simulink model "dspilbclib"  (R2020a)
settings: Solver=FixedStepDiscrete  StartTime=0.0  StopTime=inf  RelTol=1e-3  EnableMultiTasking=on
InitFcn:
  | ilbcDatatype = get_param([bdroot '/Configuration'],'ilbcDialogDatatype');
  | if strcmp(get_param([bdroot '/Configuration'],'ilbcDialogMode'), '13.33 kbit/sec mode')
  |   ilbcMode = 1;
  | else
  |   ilbcMode = 2;
  | end
model workspace: external: MAT-File dspilbcdata.mat (data not in the file)
undefined symbols (not defined in the file or in its folder): ilbc, Newton, Raphson
libraries: simulink x33, dspmtrx3 x28, dspquant2 x9, dspilbclib x8, dspstat3 x8, dspsigops x7, simulink_need_slupdate x3, dspsrcs4 x2, dspsnks4 x1, dspvision x1, dspmisc x1, dsplp x1
(part 1 of 3)
CloseFcn:
  | clear ilbcMode;
  | clear ilbcDatatype
settings Model: ExtModeAutoUpdateStatusClock=off  Creator=The MathWorks, Inc.  LastModifiedBy=Bs Computer
settings DataIOCC: LimitDataPoints=on  SaveFormat=Array  SaveOutput=off  SignalLogging=off  SaveTime=off  ReturnWorkspaceOutputs=off
settings OptimizationCC: DefaultParameterBehavior=Inlined  ExpressionDepthLimit=2147483647  InitFltsAndDblsToZero=on  EfficientFloat2IntCast=on  EfficientMapNaN2IntZero=off  LifeSpan=inf  SimCompilerOptimization=on
settings DebuggingCC: UnderspecifiedInitializationDetection=Classic  MergeDetectMultiDrivingBlocksExec=none  SolverPrmCheckMsg=warning  InheritedTsInSrcMsg=none  SigSpecEnsureSampleTimeMsg=none  Int32ToFloatConvMsg=none  ParameterPrecisionLossMsg=none  FcnCallInpInsideContextMsg=warning  AllowSymbolicDim=off  StateNameClashWarn=warning  StrictBusMsg=ErrorOnBusTreatedAsVector  SFUnexpectedBacktrackingDiag=warning  SFNoUnconditionalDefaultTransitionDiag=warning  SFExecutionAtInitializationDiag=none  ArithmeticOperatorsInVariantConditions=warning
settings HardwareCC: ProdBitPerPointer=32  ProdBitPerSizeT=32  ProdBitPerPtrDiffT=32  ProdLargestAtomicFloat=None  ProdIntDivRoundTo=Floor  ProdEndianess=Unspecified  ProdWordSize=32  ProdHWDeviceType=32-bit Generic
settings ModelReferenceCC: UpdateModelReferenceTargets=IfOutOfDate  PropagateSignalLabelsOutOfModel=off
settings SFSimCC: SimUseLocalCustomCode=off  SimParseCustomCode=off  CustomCodeUndefinedFunction=UseInterfaceOnly
settings RTWCC: RTWUseLocalCustomCode=off
settings CodeAppCC: StateflowObjectComments=on
settings GRTTargetCC: TargetFcnLib=ansi_tfl_tmw_new.mat  TargetLangStandard=C89/C90 (ANSI)  CombineOutputUpdateFcns=off  GRTInterface=on
settings ConfigComp: CovMetricSettings=dw  CovHtmlReporting=on  CovSaveCumulativeToWorkspaceVar=on  CovSaveSingleToWorkspaceVar=on  CovExternalEMLEnable=off  CovSFcnEnable=off

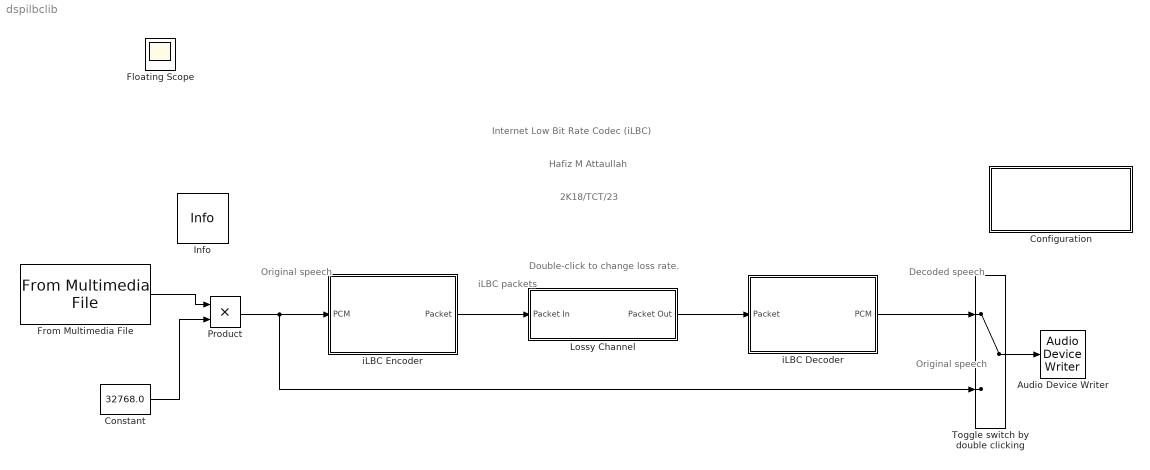
== system dspilbclib ==
  note: Internet Low Bit Rate Codec (iLBC)
  note: Original
      | speech
  note: iLBC
      | packets
  note: Double-click to change loss rate.
  note: Decoded
      | speech
  note: Original
      | speech
  note: 2K18/TCT/23
  note: Hafiz M Attaullah
  Audio Device Writer : dspsnks4/Audio Device Writer  Driver=DirectSound  Device=Default  InheritSampleRate=on  SampleRate=44100  BitDepth=16-bit integer  BufferSize=4096  NumBuffers=10  DefaultOutputChannelMapping=on  OutputChannelMapping=1:2  OutputNumUnderrunSamples=off  DriverIdx=1  DeviceWarnFlag=''
  Configuration : Subsystem  mask(iLBC Configuration){ilbcDialogMode=13.33 kbit/sec mode, ilbcDialogDatatype=double}
      mask prompts: ilbcDialogMode "iLBC mode:"; ilbcDialogDatatype "Internal data type:"
      mask help:
      | The iLBC standard is defined for two data rates: 13.33 kbit/sec and 15.20 kbit/sec.  Running under 13.33 kbit/sec, the encoder creates and outputs a compressed speech packet every 30ms.  With the 15.20 kbit/sec data rate, the encoder will output a packet every 20ms.  For the 13.33 kbit/sec mode, the packet size is a uint8 column vector of length 50, where each element represents one byte.  For the 15.20 kbit/sec mode, the packet is of length 38 bytes.
      |
      | The "Internal Data Type" option controls the precision for all internal floating point calculations in the iLBC Encoder and Decoder. The possible options are double and single precision.
      mask init:
      | if ilbcDialogMode == 1
      |     ilbcModeStr = '13.33';
      | elseif ilbcDialogMode == 2
      |     ilbcModeStr = '15.20';
      | end
      | 
      | if ilbcDialogDatatype == 1
      |     ilbcDatatype = 'double';
      | elseif ilbcDialogDatatype == 2
      |     ilbcDatatype = 'single';
      | end
      mask TypeOptions ilbcDialogMode: 13.33 kbit/sec mode | 15.20 kbit/sec mode
      mask TypeOptions ilbcDialogDatatype: double | single
      mask Display:
      | disp([ilbcModeStr ' kb/sec mode\n' ...
      |     'Internal data type: ' ilbcDatatype '\n' ...
      |     '[Double-click to change]']);
  Constant : Constant  Value=32768.0
  From Multimedia File : dspvision/From Multimedia File  inputFilename=speech_dft_8kHz.wav  readRange=[1 Inf]  loop=on  numPlays=inf  outputStreams=Audio only  videoDataType=single  audioDataType=double  inheritSampleTime=on  userDefinedSampleTime=1/30  noAudioOutput=off  isIntensityVideo=off  fourcc=RGB  colorVideoFormat=Separate color signals  outputEOF=off  dataOrg=Column-major  audioFrameSize=ilbc.BLOCKL{ilbcMode}  computeAudioFrameSize=off  outSamplingMode=Sample based
  Info : dspmisc/Info  SystemSampleTime=-1  Latency=0  AutoFrameSizeCalculation=off
      settings: SourceProductBaseCode=DS
  Lossy Channel : Subsystem  TreatAsAtomicUnit=on  mask(Lossy Channel){PercentLoss=3}
      mask prompts: PercentLoss "Percent of Packets Lost (0-100)"
      mask help:
      | This subsystem simulates a lossy channel by setting a specified percentage of packets to all zeros.  Enter the percentage of packets to be lost as a number in the range 0-100.
      |
      | Note that the packet loss concealment algorithm in the iLBC Decoder is tuned for packet loss rates between 0-10%.  Loss rates above 10% will result in decoded speech with clearly audible errors.
      mask Display: disp([num2str(PercentLoss) '% Random Packet Loss']);
  Product : Product  OutDataTypeStr=int16
  Toggle switch by double clicking : ManualSwitch
  iLBC Decoder : Subsystem  TreatAsAtomicUnit=on
  iLBC Encoder : Subsystem  TreatAsAtomicUnit=on
  Floating Scope : Scope
  wires:
  iLBC Encoder/1(Packet) -> Lossy Channel/1(Packet In)
  Toggle switch by double clicking/1 -> Audio Device Writer/1
  Lossy Channel/1(Packet Out) -> iLBC Decoder/1(Packet)
  iLBC Decoder/1(PCM) -> Toggle switch by double clicking/1
  Constant/1 -> Product/2
  From Multimedia File/1 -> Product/1
  Product/1 -> Toggle switch by double clicking/2, iLBC Encoder/1(PCM)

== system dspilbclib/Configuration ==

== system dspilbclib/Lossy Channel ==
  Packet In : Inport
  Compare To Constant : simulink/Logic and Bit Operations/Compare To Constant  relop=>  const=PercentLoss  OutDataTypeStr=uint8  ZeroCross=off
  Gain : Gain  Gain=0  OutDataTypeStr=Inherit: Same as input
  Multiport Switch : MultiPortSwitch  DataPortOrder=Zero-based contiguous  Inputs=2  zeroidx=on
  Random Source : dspsrcs4/Random Source  SrcType=Uniform  NormMethod=Ziggurat  CltLength=12  MinVal=0  MaxVal=100  MeanVal=0  VarVal=1  RepMode=Not repeatable  rawSeed=1  IsInherit=off  SampMode=Discrete  SampTime=-1  SampFrame=1  DataType=Single  OutComplex=Real  OutputFrames=on
  Packet Out : Outport
  wires:
  Multiport Switch/1 -> Packet Out/1
  Random Source/1 -> Compare To Constant/1
  Compare To Constant/1 -> Multiport Switch/1
  Packet In/1 -> Multiport Switch/3, Gain/1
  Gain/1 -> Multiport Switch/2

== system dspilbclib/iLBC Decoder ==
  note: Section 4 of the iLBC standard
  Packet : Inport
  Data Type Duplicate : DataTypeDuplicate
  Data Type Duplicate1 : DataTypeDuplicate
  Data Type Conversion : DataTypeConversion  OutDataTypeStr=int16  SaturateOnIntegerOverflow=on
  Decode Sub-Blocks (4.1 - 4.4) : Subsystem
  Delay1 : Delay  DelayLength=1  InitialCondition=0
  Delay2 : Delay  DelayLength=1  InitialCondition=0
  Enable PLC : Constant  OutDataTypeStr=boolean
  High Pass Filter (4.8) : DiscreteFilter  Numerator=ilbc.hpo_zero_coefsTbl  Denominator=ilbc.hpo_pole_coefsTbl  InputProcessing=Columns as channels (frame based)  FilterStructure=Direct form II transposed  a0EqualsOne=on  NumAccumDataTypeStr=Inherit: Same as product output  DenAccumDataTypeStr=Inherit: Same as product output
  Logical Operator : Logic  AllPortsSameDT=off  OutDataTypeStr=boolean
  Logical Operator1 : Logic  Operator=NOT  AllPortsSameDT=off  OutDataTypeStr=boolean
  Multiport Switch : MultiPortSwitch  DataPortOrder=Zero-based contiguous  Inputs=2  zeroidx=on
  Multiport Switch1 : MultiPortSwitch  DataPortOrder=Zero-based contiguous  Inputs=2  zeroidx=on
  Packet Loss Concealment (4.5) : Subsystem
  Saturation : Saturate  UpperLimit=32767  LowerLimit=-32768
  Set data type to back-propagate : Constant  OutDataTypeStr=ilbcDatatype
  Split Packet (3.8) : Subsystem  TreatAsAtomicUnit=on
  Synthesis Filtering (4.7) : Subsystem  TreatAsAtomicUnit=on
  PCM : Outport
  wires:
  Enable PLC/1 -> Logical Operator/2
  Set data type to back-propagate/1 -> Data Type Duplicate/1
  Logical Operator1/1 -> Logical Operator/1
  Logical Operator/1 -> Packet Loss Concealment (4.5)/Enable
  Packet Loss Concealment (4.5)/2(Synthesis) -> Multiport Switch1/2
  Packet Loss Concealment (4.5)/1(Residual) -> Multiport Switch/2
  Decode Sub-Blocks (4.1 - 4.4)/2(Synthesis) -> Data Type Duplicate1/2, Multiport Switch1/3
  Decode Sub-Blocks (4.1 - 4.4)/1(Residual) -> Multiport Switch/3
  Split Packet (3.8)/8(Good Frame) -> Decode Sub-Blocks (4.1 - 4.4)/Enable, Multiport Switch1/1, Multiport Switch/1, Logical Operator1/1
  Split Packet (3.8)/1(Lsf Indices) -> Decode Sub-Blocks (4.1 - 4.4)/1(Lsf Indices)
  Split Packet (3.8)/7(Gain Indices) -> Decode Sub-Blocks (4.1 - 4.4)/7(Gain Indices)
  Split Packet (3.8)/6(Code Indices) -> Decode Sub-Blocks (4.1 - 4.4)/6(Code Indices)
  Split Packet (3.8)/5(Start State Indices) -> Decode Sub-Blocks (4.1 - 4.4)/5(Start State Indices)
  Split Packet (3.8)/4(Start State Gain Index) -> Decode Sub-Blocks (4.1 - 4.4)/4(Start State Gain Index)
  Split Packet (3.8)/3(State First) -> Decode Sub-Blocks (4.1 - 4.4)/3(State First)
  Split Packet (3.8)/2(Start State Number) -> Decode Sub-Blocks (4.1 - 4.4)/2(Start State Number)
  Synthesis Filtering (4.7)/1(Decoded Block) -> High Pass Filter (4.8)/1
  Saturation/1 -> Data Type Duplicate/2, Data Type Conversion/1
  Data Type Conversion/1 -> PCM/1
  Packet/1 -> Split Packet (3.8)/1(Packet)
  High Pass Filter (4.8)/1 -> Saturation/1
  Multiport Switch/1 -> Delay1/1, Synthesis Filtering (4.7)/1(Residual)
  Delay1/1 -> Packet Loss Concealment (4.5)/1(Last Residual)
  Multiport Switch1/1 -> Delay2/1, Data Type Duplicate1/1, Synthesis Filtering (4.7)/2(Synthesis Filters)
  Delay2/1 -> Packet Loss Concealment (4.5)/2(Last Synthesis)

== system dspilbclib/iLBC Encoder ==
  note: Section 3 of the iLBC standard
  PCM : Inport
  Calculate Residual (3.3) : Subsystem  TreatAsAtomicUnit=on
  Create Packet (3.8) : Subsystem  TreatAsAtomicUnit=on
  Data Type Conversion : DataTypeConversion  OutDataTypeStr=ilbcDatatype
  Encode Data (3.5 - 3.7) : Subsystem  TreatAsAtomicUnit=on
  Encoder LPC Analysis (3.2) : Subsystem  TreatAsAtomicUnit=on
  High Pass (3.1) : DiscreteFilter  Numerator=ilbc.hpi_zero_coefsTbl  Denominator=ilbc.hpi_pole_coefsTbl  InputProcessing=Columns as channels (frame based)  FilterStructure=Direct form II transposed  a0EqualsOne=on  NumAccumDataTypeStr=Inherit: Same as product output  DenAccumDataTypeStr=Inherit: Same as product output
  Perceptual Weighting (3.4) : dspmtrx3/Array-Vector Multiply  mode=Mute  saveAsFlag=0  Dimension=1  V_Source=Dialog parameter  V_VectFromMask=ilbc.LPC_CHIRP_WEIGHTDENUM.^(0:10)'  roundingMode=Floor  overflowMode=off  firstCoeffSignedness=Auto  firstCoeffDataTypeStr=Inherit: Same word length as input  firstCoeffMin=[]  firstCoeffMax=[]  firstCoeffLastDataTypeStr=Inherit: Same word length as input  prodOutputSignedness=Auto  accumSignedness=Auto  outputSignedness=Auto  outputDataTypeStr=Inherit: Same as product output  outputMin=[]  outputMax=[]  outputLastDataTypeStr=Inherit: Same as product output
      settings: SourceProductBaseCode=DS
  Packet : Outport
  wires:
  Data Type Conversion/1 -> High Pass (3.1)/1
  Encoder LPC Analysis (3.2)/1(LSF Indices) -> Create Packet (3.8)/1(LSF Indices)
  High Pass (3.1)/1 -> Calculate Residual (3.3)/2(Data), Encoder LPC Analysis (3.2)/1(Data)
  Encode Data (3.5 - 3.7)/6(Gain Indices) -> Create Packet (3.8)/7(Gain Indices)
  Encode Data (3.5 - 3.7)/5(Code Indices) -> Create Packet (3.8)/6(Code Indices)
  Encode Data (3.5 - 3.7)/4(Start State Indices) -> Create Packet (3.8)/5(Start State Indices)
  Encode Data (3.5 - 3.7)/3(Start State Gain Index) -> Create Packet (3.8)/4(Start State Gain Index)
  Encode Data (3.5 - 3.7)/2(State First) -> Create Packet (3.8)/3(State First)
  Encode Data (3.5 - 3.7)/1(Start State Number) -> Create Packet (3.8)/2(Start State Number)
  Encoder LPC Analysis (3.2)/3(Weight Filters) -> Perceptual Weighting (3.4)/1
  Calculate Residual (3.3)/1(Residual) -> Encode Data (3.5 - 3.7)/3(Residual)
  Create Packet (3.8)/1(Packet) -> Packet/1
  PCM/1 -> Data Type Conversion/1
  Perceptual Weighting (3.4)/1 -> Encode Data (3.5 - 3.7)/2(Weights)
  Encoder LPC Analysis (3.2)/2(Synthesis Filters) -> Calculate Residual (3.3)/1(Synthesis Filters), Encode Data (3.5 - 3.7)/1(Synthesis)

== system dspilbclib/iLBC Decoder/Decode Sub-Blocks (4.1 - 4.4) ==
  Lsf Indices : Inport
  Start State Number : Inport  Port=2
  State First : Inport  Port=3
  Start State Gain Index : Inport  Port=4
  Start State Indices : Inport  Port=5
  Code Indices : Inport  Port=6
  Gain Indices : Inport  Port=7
  Enable : EnablePort
  Decode Remaining Sub-Blocks (4.3 - 4.4) : Subsystem  TreatAsAtomicUnit=on
  Decode Start State : dspilbclib/Decode Start State  SystemSampleTime=-1  Latency=0  AutoFrameSizeCalculation=off
      settings: SourceProductBaseCode=DS
  Decoder LPC Analysis (4.1) : Subsystem  TreatAsAtomicUnit=on
  Selector1 : Selector  NumberOfDimensions=2  InputPortWidth=3  IndexOptions=Select all,Index vector (port)  Indices=-1,-1  OutputSizes=1
  Residual : Outport
  Synthesis : Outport  Port=2
  wires:
  Decode Start State/1 -> Decode Remaining Sub-Blocks (4.3 - 4.4)/1(Initial Codebook)
  Start State Number/1 -> Selector1/2, Decode Remaining Sub-Blocks (4.3 - 4.4)/4(Start State Number)
  Selector1/1 -> Decode Start State/3
  State First/1 -> Decode Start State/4, Decode Remaining Sub-Blocks (4.3 - 4.4)/5(State First)
  Lsf Indices/1 -> Decoder LPC Analysis (4.1)/1(LSF Indices)
  Decoder LPC Analysis (4.1)/1(Synthesis) -> Synthesis/1, Selector1/1
  Start State Indices/1 -> Decode Start State/1
  Start State Gain Index/1 -> Decode Start State/2
  Code Indices/1 -> Decode Remaining Sub-Blocks (4.3 - 4.4)/2(Code Indices)
  Gain Indices/1 -> Decode Remaining Sub-Blocks (4.3 - 4.4)/3(Gain Indices)
  Decode Remaining Sub-Blocks (4.3 - 4.4)/1(Residual) -> Residual/1

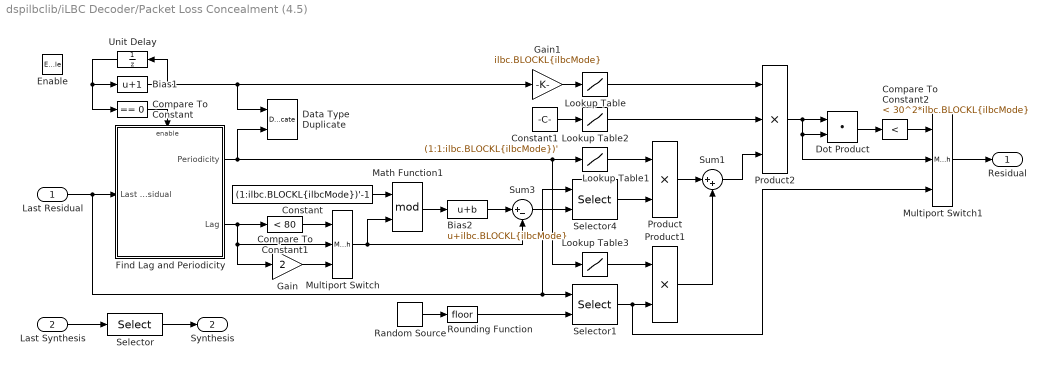
== system dspilbclib/iLBC Decoder/Packet Loss Concealment (4.5) ==
  Last Residual : Inport
  Last Synthesis : Inport  Port=2
  Enable : EnablePort  StatesWhenEnabling=reset
  Bias1 : Bias  Bias=1
  Bias2 : Bias  Bias=ilbc.BLOCKL{ilbcMode}
  Compare To Constant : simulink/Logic and Bit Operations/Compare To Constant  relop===  const=0  OutDataTypeStr=boolean  ZeroCross=off
  Compare To Constant1 : simulink/Logic and Bit Operations/Compare To Constant  relop=<  const=80  OutDataTypeStr=uint8  ZeroCross=off
  Compare To Constant2 : simulink/Logic and Bit Operations/Compare To Constant  relop=<  const=30^2*ilbc.BLOCKL{ilbcMode}  OutDataTypeStr=boolean  ZeroCross=off
  Constant : Constant  Value=(1:ilbc.BLOCKL{ilbcMode})'-1  VectorParams1D=off  OutDataTypeStr=Inherit: Inherit via back propagation
  Constant1 : Constant  Value=(1:1:ilbc.BLOCKL{ilbcMode})'  VectorParams1D=off  OutDataTypeStr=Inherit: Inherit via back propagation
  Data Type Duplicate : DataTypeDuplicate
  Dot Product : DotProduct  InputSameDT=on  OutDataTypeStr=Inherit: Inherit via internal rule
  Find Lag and Periodicity : Subsystem  TreatAsAtomicUnit=on
  Gain : Gain  Gain=2  OutDataTypeStr=Inherit: Same as input
  Gain1 : Gain  Gain=ilbc.BLOCKL{ilbcMode}  OutDataTypeStr=Inherit: Inherit via back propagation  ParamDataTypeStr=Inherit: Same as input
  Lookup Table : Lookup_n-D  NumberOfTableDimensions=1  BreakpointsForDimension1=[0 320 640 960 1280]  Table=[1.0 0.9 0.7 0.5 0.0]  InterpMethod=Flat  InputSameDT=on
  Lookup Table1 : Lookup_n-D  NumberOfTableDimensions=1  BreakpointsForDimension1=[0.3 0.6]  Table=[0 1]  ExtrapMethod=Clip  InputSameDT=on
  Lookup Table2 : Lookup_n-D  NumberOfTableDimensions=1  BreakpointsForDimension1=[80 160 240]  Table=[1.00 0.95 0.90]  ExtrapMethod=Clip  InputSameDT=on
  Lookup Table3 : Lookup_n-D  NumberOfTableDimensions=1  BreakpointsForDimension1=[0.3 0.6]  Table=[1 0]  ExtrapMethod=Clip  InputSameDT=on
  Math Function1 : Math  Operator=mod  SignedPower=on  SaturateOnIntegerOverflow=on
  Multiport Switch : MultiPortSwitch  DataPortOrder=Zero-based contiguous  Inputs=2  zeroidx=on
  Multiport Switch1 : MultiPortSwitch  DataPortOrder=Zero-based contiguous  Inputs=2  zeroidx=on
  Product : Product  RndMeth=Zero
  Product1 : Product  RndMeth=Zero
  Product2 : Product  Inputs=3  RndMeth=Zero  OutDataTypeStr=Inherit: Same as first input
  Random Source : dspsrcs4/Random Source  SrcType=Uniform  NormMethod=Ziggurat  CltLength=12  MinVal=ilbc.BLOCKL{ilbcMode}-70  MaxVal=ilbc.BLOCKL{ilbcMode}-0.001  MeanVal=0  VarVal=1  RepMode=Not repeatable  rawSeed=1  IsInherit=off  SampMode=Discrete  SampTime=-1  SampFrame=ilbc.BLOCKL{ilbcMode}  DataType=Single  OutComplex=Real  OutputFrames=off
  Rounding Function : Rounding
  Selector : Selector  NumberOfDimensions=2  InputPortWidth=3  IndexOptions=Select all,Index vector (dialog)  Indices=[1 3],repmat(ilbc.NSUB{ilbcMode},1,ilbc.NSUB{ilbcMode})  OutputSizes=1,1
  Selector1 : Selector  NumberOfDimensions=2  IndexMode=Zero-based  InputPortWidth=3  IndexOptions=Index vector (port),Select all  Indices=[1 3],1  OutputSizes=1,1
  Selector4 : Selector  NumberOfDimensions=2  IndexMode=Zero-based  InputPortWidth=3  IndexOptions=Index vector (port),Select all  Indices=[1 3],1  OutputSizes=1,1
  Sum1 : Sum  Inputs=|++
  Sum3 : Sum  Inputs=|+-
  Unit Delay : UnitDelay  SampleTime=-1  HasFrameUpgradeWarning=on
  Residual : Outport
  Synthesis : Outport  Port=2
  wires:
  Bias1/1 -> Data Type Duplicate/1, Gain1/1, Unit Delay/1
  Rounding Function/1 -> Selector1/2
  Unit Delay/1 -> Compare To Constant/1, Bias1/1
  Compare To Constant/1 -> Find Lag and Periodicity/Enable
  Random Source/1 -> Rounding Function/1
  Gain/1 -> Multiport Switch/3
  Product1/1 -> Sum1/2
  Product/1 -> Sum1/1
  Selector1/1 -> Multiport Switch1/3, Product1/2
  Lookup Table3/1 -> Product1/1
  Selector4/1 -> Product/2
  Lookup Table1/1 -> Product/1
  Multiport Switch/1 -> Sum3/2, Math Function1/2
  Sum3/1 -> Selector4/2
  Bias2/1 -> Sum3/1
  Math Function1/1 -> Bias2/1
  Constant/1 -> Math Function1/1
  Product2/1 -> Multiport Switch1/2, Dot Product/2, Dot Product/1
  Last Residual/1 -> Selector1/1, Selector4/1, Find Lag and Periodicity/1(Last Residual)
  Lookup Table2/1 -> Product2/2
  Lookup Table/1 -> Product2/1
  Multiport Switch1/1 -> Residual/1
  Compare To Constant2/1 -> Multiport Switch1/1
  Dot Product/1 -> Compare To Constant2/1
  Sum1/1 -> Product2/3
  Constant1/1 -> Lookup Table2/1
  Gain1/1 -> Lookup Table/1
  Compare To Constant1/1 -> Multiport Switch/1
  Find Lag and Periodicity/1(Periodicity) -> Data Type Duplicate/2, Lookup Table3/1, Lookup Table1/1
  Find Lag and Periodicity/2(Lag) -> Gain/1, Multiport Switch/2, Compare To Constant1/1
  Selector/1 -> Synthesis/1
  Last Synthesis/1 -> Selector/1

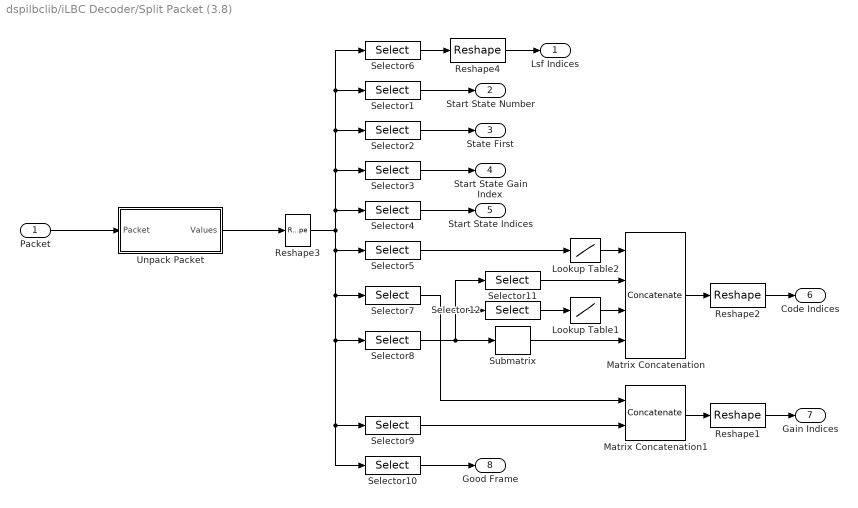
== system dspilbclib/iLBC Decoder/Split Packet (3.8) ==
  Packet : Inport
  Lookup Table1 : Lookup_n-D  NumberOfTableDimensions=1  BreakpointsForDimension1=[0:255]  Table=[0:43 108:171 236:255 zeros(1,128)]  ExtrapMethod=Clip  InputSameDT=on
  Lookup Table2 : Lookup_n-D  NumberOfTableDimensions=1  BreakpointsForDimension1=[0:255]  Table=[0:57 zeros(1,6) 128:185 zeros(1,134)]  ExtrapMethod=Clip  InputSameDT=on
  Matrix Concatenation : Concatenate  NumInputs=4  Mode=Multidimensional array
  Matrix Concatenation1 : Concatenate  Mode=Multidimensional array
  Reshape1 : Reshape  OutputDimensionality=Customize  OutputDimensions=[3 (ilbc.NSUB{ilbcMode}-1)]
  Reshape2 : Reshape  OutputDimensionality=Customize  OutputDimensions=[3 (ilbc.NSUB{ilbcMode}-1)]
  Reshape3 : Reshape  OutputDimensionality=Column vector (2-D)
  Reshape4 : Reshape  OutputDimensionality=Customize  OutputDimensions=[3 (3-ilbcMode)]
  Selector1 : Selector  NumberOfDimensions=2  InputPortWidth=3  IndexOptions=Index vector (dialog),Select all  Indices=ilbc.packet_idxTbl{ilbcMode}{2},-1  OutputSizes=1
  Selector10 : Selector  NumberOfDimensions=2  InputPortWidth=3  IndexOptions=Index vector (dialog),Select all  Indices=ilbc.packet_idxTbl{ilbcMode}{10},-1  OutputSizes=1
  Selector11 : Selector  NumberOfDimensions=2  InputPortWidth=3  IndexOptions=Index vector (dialog),Select all  Indices=1,-1  OutputSizes=1
  Selector12 : Selector  NumberOfDimensions=2  InputPortWidth=3  IndexOptions=Index vector (dialog),Select all  Indices=2:3,-1  OutputSizes=1
  Selector2 : Selector  NumberOfDimensions=2  InputPortWidth=3  IndexOptions=Index vector (dialog),Select all  Indices=ilbc.packet_idxTbl{ilbcMode}{3},-1  OutputSizes=1
  Selector3 : Selector  NumberOfDimensions=2  InputPortWidth=3  IndexOptions=Index vector (dialog),Select all  Indices=ilbc.packet_idxTbl{ilbcMode}{4},-1  OutputSizes=1
  Selector4 : Selector  NumberOfDimensions=2  InputPortWidth=3  IndexOptions=Index vector (dialog),Select all  Indices=ilbc.packet_idxTbl{ilbcMode}{5},-1  OutputSizes=1
  Selector5 : Selector  NumberOfDimensions=2  InputPortWidth=3  IndexOptions=Index vector (dialog),Select all  Indices=ilbc.packet_idxTbl{ilbcMode}{6},-1  OutputSizes=1
  Selector6 : Selector  NumberOfDimensions=2  InputPortWidth=3  IndexOptions=Index vector (dialog),Select all  Indices=ilbc.packet_idxTbl{ilbcMode}{1},-1  OutputSizes=1
  Selector7 : Selector  NumberOfDimensions=2  InputPortWidth=3  IndexOptions=Index vector (dialog),Select all  Indices=ilbc.packet_idxTbl{ilbcMode}{7},-1  OutputSizes=1
  Selector8 : Selector  NumberOfDimensions=2  InputPortWidth=3  IndexOptions=Index vector (dialog),Select all  Indices=ilbc.packet_idxTbl{ilbcMode}{8},-1  OutputSizes=1
  Selector9 : Selector  NumberOfDimensions=2  InputPortWidth=3  IndexOptions=Index vector (dialog),Select all  Indices=ilbc.packet_idxTbl{ilbcMode}{9},-1  OutputSizes=1
  Submatrix : dspmtrx3/Submatrix  RowSpan=Range of rows  RowStartMode=Index  RowStartIndex=4  RowEndMode=Last  RowEndIndex=1  ColSpan=All columns  ColStartMode=First  ColStartIndex=1  ColEndMode=Last  ColEndIndex=1
  Unpack Packet : Subsystem  TreatAsAtomicUnit=on
  Lsf Indices : Outport
  Start State Number : Outport  Port=2
  State First : Outport  Port=3
  Start State Gain Index : Outport  Port=4
  Start State Indices : Outport  Port=5
  Code Indices : Outport  Port=6
  Gain Indices : Outport  Port=7
  Good Frame : Outport  Port=8
  wires:
  Unpack Packet/1(Values) -> Reshape3/1
  Packet/1 -> Unpack Packet/1(Packet)
  Lookup Table1/1 -> Matrix Concatenation/3
  Lookup Table2/1 -> Matrix Concatenation/1
  Selector12/1 -> Lookup Table1/1
  Selector11/1 -> Matrix Concatenation/2
  Submatrix/1 -> Matrix Concatenation/4
  Selector8/1 -> Submatrix/1, Selector12/1, Selector11/1
  Selector5/1 -> Lookup Table2/1
  Reshape4/1 -> Lsf Indices/1
  Reshape3/1 -> Selector1/1, Selector6/1, Selector2/1, Selector3/1, Selector4/1, Selector5/1, Selector7/1, Selector9/1, Selector10/1, Selector8/1
  Selector6/1 -> Reshape4/1
  Selector10/1 -> Good Frame/1
  Selector7/1 -> Matrix Concatenation1/1
  Selector9/1 -> Matrix Concatenation1/2
  Selector2/1 -> State First/1
  Selector4/1 -> Start State Indices/1
  Selector3/1 -> Start State Gain Index/1
  Selector1/1 -> Start State Number/1
  Reshape1/1 -> Gain Indices/1
  Reshape2/1 -> Code Indices/1
  Matrix Concatenation1/1 -> Reshape1/1
  Matrix Concatenation/1 -> Reshape2/1

== system dspilbclib/iLBC Decoder/Synthesis Filtering (4.7) ==
  Residual : Inport
  Synthesis Filters : Inport  Port=2
  Assignment : Assignment  NumberOfDimensions=2  OutputInitialize=Specify size for each dimension in table  IndexOptions=Assign all,Index vector (port)  Indices=-1,1  OutputSizes=40,ilbc.NSUB{ilbcMode}
  For Iterator : ForIterator  IterationLimit=ilbc.NSUB{ilbcMode}  IterationVariableDataType=int8
  Reshape : Reshape  OutputDimensionality=Customize  OutputDimensions=[40 ilbc.NSUB{ilbcMode}]
  Reshape1 : Reshape  OutputDimensionality=Column vector (2-D)  OutputDimensions=[50 4]
  Selector1 : Selector  NumberOfDimensions=2  InputPortWidth=3  IndexOptions=Select all,Index vector (port)  Indices=-1,-1  OutputSizes=1
  Selector2 : Selector  NumberOfDimensions=2  InputPortWidth=3  IndexOptions=Select all,Index vector (port)  Indices=-1,-1  OutputSizes=1
  Time-Varying Analysis Filter3 : AllpoleFilter  CoefSource=Input port  AccumDataTypeStr=Inherit: Same as product output
      settings: InputPortMap=u0,u1
  tp22016052_e266_46f3_948b_11691b873d03 : Math  Operator=transpose  SignedPower=on  SaturateOnIntegerOverflow=on
  Decoded Block : Outport
  wires:
  Reshape1/1 -> Decoded Block/1
  Assignment/1 -> Reshape1/1
  Time-Varying Analysis Filter3/1 -> Assignment/1
  Reshape/1 -> Selector2/1
  For Iterator/1 -> Assignment/2, Selector2/2, Selector1/2
  Selector2/1 -> Time-Varying Analysis Filter3/1
  Synthesis Filters/1 -> Selector1/1
  Residual/1 -> Reshape/1
  Selector1/1 -> tp22016052_e266_46f3_948b_11691b873d03/1
  tp22016052_e266_46f3_948b_11691b873d03/1 -> Time-Varying Analysis Filter3/2

== system dspilbclib/iLBC Encoder/Calculate Residual (3.3) ==
  Synthesis Filters : Inport
  Data : Inport  Port=2
  Assignment1 : Assignment  NumberOfDimensions=2  OutputInitialize=Specify size for each dimension in table  IndexOptions=Assign all,Index vector (port)  Indices=-1,1  OutputSizes=40,ilbc.NSUB{ilbcMode}
  For Iterator : ForIterator  IterationLimit=ilbc.NSUB{ilbcMode}  IterationVariableDataType=int8
  Reshape2 : Reshape  OutputDimensionality=Customize  OutputDimensions=[40 ilbc.NSUB{ilbcMode}]
  Selector1 : Selector  NumberOfDimensions=2  InputPortWidth=3  IndexOptions=Select all,Index vector (port)  Indices=-1,-1  OutputSizes=1
  Selector2 : Selector  NumberOfDimensions=2  InputPortWidth=3  IndexOptions=Select all,Index vector (port)  Indices=-1,-1  OutputSizes=1
  Time-Varying Analysis Filter1 : DiscreteFir  CoefSource=Input port  Coefficients=[1 -.95]  InputProcessing=Columns as channels (frame based)  AccumDataTypeStr=Inherit: Same as product output  OutDataTypeStr=Inherit: Same as input
      settings: InputPortMap=u0,u1
  tp7f274a0e_53ba_403c_9211_c5fc596ffe5e : Math  Operator=transpose  SignedPower=on  SaturateOnIntegerOverflow=on
  Residual : Outport
  wires:
  Time-Varying Analysis Filter1/1 -> Assignment1/1
  Selector2/1 -> Time-Varying Analysis Filter1/1
  Assignment1/1 -> Residual/1
  Synthesis Filters/1 -> Selector1/1
  Data/1 -> Reshape2/1
  Reshape2/1 -> Selector2/1
  For Iterator/1 -> Selector1/2, Selector2/2, Assignment1/2
  Selector1/1 -> tp7f274a0e_53ba_403c_9211_c5fc596ffe5e/1
  tp7f274a0e_53ba_403c_9211_c5fc596ffe5e/1 -> Time-Varying Analysis Filter1/2

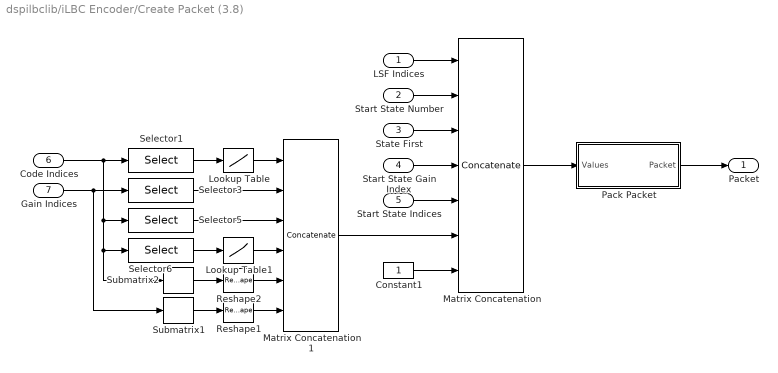
== system dspilbclib/iLBC Encoder/Create Packet (3.8) ==
  LSF Indices : Inport
  Start State Number : Inport  Port=2
  State First : Inport  Port=3
  Start State Gain Index : Inport  Port=4
  Start State Indices : Inport  Port=5
  Code Indices : Inport  Port=6
  Gain Indices : Inport  Port=7
  Constant1 : Constant  OutDataTypeStr=uint8
  Lookup Table : Lookup_n-D  NumberOfTableDimensions=1  BreakpointsForDimension1=[0:255]  Table=[0:57 zeros(1,70) 64:121 zeros(1,70)]  ExtrapMethod=Clip  InputSameDT=on
  Lookup Table1 : Lookup_n-D  NumberOfTableDimensions=1  BreakpointsForDimension1=[0:255]  Table=[0:43 zeros(1,64) 44:107 zeros(1,64) 108:127]  ExtrapMethod=Clip  InputSameDT=on
  Matrix Concatenation : Concatenate  NumInputs=7  Mode=Multidimensional array
  Matrix Concatenation1 : Concatenate  NumInputs=6  Mode=Multidimensional array
  Pack Packet : Subsystem  TreatAsAtomicUnit=on
  Reshape1 : Reshape  OutputDimensionality=Column vector (2-D)
  Reshape2 : Reshape  OutputDimensionality=Column vector (2-D)
  Selector1 : Selector  NumberOfDimensions=2  InputPortWidth=3  IndexOptions=Select all,Index vector (dialog)  Indices=-1,1  OutputSizes=1
  Selector3 : Selector  NumberOfDimensions=2  InputPortWidth=3  IndexOptions=Select all,Index vector (dialog)  Indices=-1,1  OutputSizes=1
  Selector5 : Selector  NumberOfDimensions=2  InputPortWidth=3  IndexOptions=Index vector (dialog),Index vector (dialog)  Indices=1,2  OutputSizes=1
  Selector6 : Selector  NumberOfDimensions=2  InputPortWidth=3  IndexOptions=Index vector (dialog),Index vector (dialog)  Indices=2:3,2  OutputSizes=1
  Submatrix1 : dspmtrx3/Submatrix  RowSpan=All rows  RowStartMode=First  RowStartIndex=1  RowEndMode=Last  RowEndIndex=1  ColSpan=Range of columns  ColStartMode=Index  ColStartIndex=2  ColEndMode=Last  ColEndIndex=1
  Submatrix2 : dspmtrx3/Submatrix  RowSpan=All rows  RowStartMode=First  RowStartIndex=1  RowEndMode=Last  RowEndIndex=1  ColSpan=Range of columns  ColStartMode=Index  ColStartIndex=3  ColEndMode=Last  ColEndIndex=1
  Packet : Outport
  wires:
  Pack Packet/1(Packet) -> Packet/1
  Matrix Concatenation/1 -> Pack Packet/1(Values)
  Lookup Table1/1 -> Matrix Concatenation1/4
  Lookup Table/1 -> Matrix Concatenation1/1
  Selector3/1 -> Matrix Concatenation1/2
  Gain Indices/1 -> Submatrix1/1, Selector3/1
  Reshape1/1 -> Matrix Concatenation1/6
  Reshape2/1 -> Matrix Concatenation1/5
  Submatrix2/1 -> Reshape2/1
  Selector5/1 -> Matrix Concatenation1/3
  Selector6/1 -> Lookup Table1/1
  Submatrix1/1 -> Reshape1/1
  Matrix Concatenation1/1 -> Matrix Concatenation/6
  Selector1/1 -> Lookup Table/1
  Code Indices/1 -> Submatrix2/1, Selector6/1, Selector5/1, Selector1/1
  Constant1/1 -> Matrix Concatenation/7
  Start State Indices/1 -> Matrix Concatenation/5
  Start State Gain Index/1 -> Matrix Concatenation/4
  State First/1 -> Matrix Concatenation/3
  Start State Number/1 -> Matrix Concatenation/2
  LSF Indices/1 -> Matrix Concatenation/1

== system dspilbclib/iLBC Encoder/Encode Data (3.5 - 3.7) ==
  Synthesis : Inport
  Weights : Inport  Port=2
  Residual : Inport  Port=3
  Decode Start State (3.5.3 last paragraph) : dspilbclib/Decode Start State  SystemSampleTime=-1  Latency=0  AutoFrameSizeCalculation=off
      settings: SourceProductBaseCode=DS
  Encode Remaining Sub-Blocks (3.6 - 3.7) : Subsystem
  Encode Start State (3.5.2 - 3.5.3) : Subsystem  TreatAsAtomicUnit=on
  Extract Sub-Blocks (3.5.1) and Sort LPC Filters : Subsystem  TreatAsAtomicUnit=on
  Start State Number : Outport
  State First : Outport  Port=2
  Start State Gain Index : Outport  Port=3
  Start State Indices : Outport  Port=4
  Code Indices : Outport  Port=5
  Gain Indices : Outport  Port=6
  wires:
  Extract Sub-Blocks (3.5.1) and Sort LPC Filters/3(Start State Number) -> Start State Number/1, Encode Remaining Sub-Blocks (3.6 - 3.7)/3(Start State Number)
  Extract Sub-Blocks (3.5.1) and Sort LPC Filters/7(Start State Synthesis) -> Decode Start State (3.5.3 last paragraph)/3, Encode Start State (3.5.2 - 3.5.3)/3(Synthesis Filter)
  Extract Sub-Blocks (3.5.1) and Sort LPC Filters/6(Start State Weights) -> Encode Start State (3.5.2 - 3.5.3)/2(Weight Filters)
  Extract Sub-Blocks (3.5.1) and Sort LPC Filters/5(Start State) -> Encode Start State (3.5.2 - 3.5.3)/1(Start State)
  Weights/1 -> Extract Sub-Blocks (3.5.1) and Sort LPC Filters/3(Weights)
  Extract Sub-Blocks (3.5.1) and Sort LPC Filters/2(Sorted Weights) -> Encode Remaining Sub-Blocks (3.6 - 3.7)/2(Weights)
  Extract Sub-Blocks (3.5.1) and Sort LPC Filters/1(Sorted Sub-blocks) -> Encode Remaining Sub-Blocks (3.6 - 3.7)/1(Sub-blocks)
  Synthesis/1 -> Extract Sub-Blocks (3.5.1) and Sort LPC Filters/2(Synthesis)
  Encode Start State (3.5.2 - 3.5.3)/2(Start State Gain Index) -> Start State Gain Index/1, Decode Start State (3.5.3 last paragraph)/2
  Decode Start State (3.5.3 last paragraph)/1 -> Encode Remaining Sub-Blocks (3.6 - 3.7)/5(Initial Codebook)
  Encode Remaining Sub-Blocks (3.6 - 3.7)/2(Gains) -> Gain Indices/1
  Encode Remaining Sub-Blocks (3.6 - 3.7)/1(Codes) -> Code Indices/1
  Encode Start State (3.5.2 - 3.5.3)/1(Start State Indices) -> Start State Indices/1, Decode Start State (3.5.3 last paragraph)/1
  Residual/1 -> Extract Sub-Blocks (3.5.1) and Sort LPC Filters/1(Residual)
  Extract Sub-Blocks (3.5.1) and Sort LPC Filters/4(State First) -> Encode Remaining Sub-Blocks (3.6 - 3.7)/4(State First), State First/1, Decode Start State (3.5.3 last paragraph)/4, Encode Start State (3.5.2 - 3.5.3)/4(State First)

== system dspilbclib/iLBC Encoder/Encoder LPC Analysis (3.2) ==
  note: 3.2.1
  note: 3.2.2
  note: 3.2.3
  Data : Inport
  Autocorrelation : dspstat3/Autocorrelation  AllPositiveLags=off  maxlag=10  bias=None  domain=Time  roundingMode=Floor  overflowMode=off  outputDataTypeStr=Inherit: Same as accumulator  outputMin=[]  outputMax=[]  outputLastDataTypeStr=Inherit: Same as accumulator
      settings: SourceProductBaseCode=DS
  Delay2 : Delay  DelayLength=1  InitialCondition=0
  Find Perceptual Weight Filters (3.2.6) : dspilbclib/Find LPC Filters  SystemSampleTime=-1  Latency=0  AutoFrameSizeCalculation=off
      settings: SourceProductBaseCode=DS
  Find Synthesis Filters (3.2.6) : dspilbclib/Find LPC Filters  SystemSampleTime=-1  Latency=0  AutoFrameSizeCalculation=off
      settings: SourceProductBaseCode=DS
  Gain : Gain  Gain=ilbc.lpc_winTbls{ilbcMode}
  LPC to LSF/LSP Conversion1 : dsplp/LPC to LSF//LSP Conversion  output=LSF in range (0 pi)  NSteps=64  NBisects=6  RootStatus=off  correction=off  lastLSP=off  error=Ignore
      settings: SourceProductBaseCode=DS
  LSF Quantization (3.2.4) : Subsystem
  Levinson-Durbin : dspsolvers/Levinson-Durbin  coeffOutFcn=OBSOLETE  coeffOutFcnActive=A  outP=off  zeroInpHandling=on  roundingMode=Floor  overflowMode=off  prodOutputMode=Binary point scaling  prodOutputWordLength=32  prodOutputFracLength=30  prodOutputDataTypeStr=fixdt(1,32,30)  prodOutputLastDataTypeStr=fixdt(1,32,30)  accumMode=Binary point scaling  accumWordLength=32  accumFracLength=30  accumDataTypeStr=fixdt(1,32,30)  accumLastDataTypeStr=fixdt(1,32,30)  firstCoeffMode=Binary point scaling  firstCoeffWordLength=16  firstCoeffFracLength=15  firstCoeffDataTypeStr=fixdt(1,16,15)  firstCoeffMin=[]  firstCoeffMax=[]  firstCoeffLastDataTypeStr=fixdt(1,16,15)  secondCoeffMode=Binary point scaling  secondCoeffWordLength=16  secondCoeffFracLength=15  secondCoeffDataTypeStr=fixdt(1,16,15)  secondCoeffMin=[]  secondCoeffMax=[]  secondCoeffLastDataTypeStr=fixdt(1,16,15)  outputMin=[]  outputMax=[]
      settings: SourceProductBaseCode=DS  allowOverrides=off
  Matrix Concatenation3 : Concatenate  Mode=Multidimensional array
  Matrix Scaling : dspmtrx3/Array-Vector Multiply  mode=Mute  saveAsFlag=0  Dimension=1  V_Source=Dialog parameter  V_VectFromMask=ilbc.lpc_lagwinTbl  roundingMode=Floor  overflowMode=off  firstCoeffSignedness=Auto  firstCoeffDataTypeStr=Inherit: Same word length as input  firstCoeffMin=[]  firstCoeffMax=[]  firstCoeffLastDataTypeStr=Inherit: Same word length as input  prodOutputSignedness=Auto  accumSignedness=Auto  outputSignedness=Auto  outputDataTypeStr=Inherit: Same as product output  outputMin=[]  outputMax=[]  outputLastDataTypeStr=Inherit: Same as product output
      settings: SourceProductBaseCode=DS
  Matrix Scaling1 : dspmtrx3/Array-Vector Multiply  mode=Mute  saveAsFlag=0  Dimension=1  V_Source=Dialog parameter  V_VectFromMask=ilbc.LPC_CHIRP_SYNTDENUM.^(0:10)'  roundingMode=Floor  overflowMode=off  firstCoeffSignedness=Auto  firstCoeffDataTypeStr=Inherit: Same word length as input  firstCoeffMin=[]  firstCoeffMax=[]  firstCoeffLastDataTypeStr=Inherit: Same word length as input  prodOutputSignedness=Auto  accumSignedness=Auto  outputSignedness=Auto  outputDataTypeStr=Inherit: Same as product output  outputMin=[]  outputMax=[]  outputLastDataTypeStr=Inherit: Same as product output
      settings: SourceProductBaseCode=DS
  Reshape : Reshape  OutputDimensionality=Customize  OutputDimensions=[240 (3-ilbcMode)]
  Selector : Selector  NumberOfDimensions=2  InputPortWidth=3  IndexOptions=Index vector (dialog),Index vector (dialog)  Indices=ilbc.lpc_winIdxTbl{ilbcMode},1  OutputSizes=1,1
  Submatrix1 : dspmtrx3/Submatrix  RowSpan=Range of rows  RowStartMode=Offset from last  RowStartIndex=ilbc.BUFFEROVERLAP{ilbcMode}-1  RowEndMode=Last  RowEndIndex=1  ColSpan=All columns  ColStartMode=Offset from last  ColStartIndex=1  ColEndMode=Last  ColEndIndex=1
  LSF Indices : Outport
  Synthesis Filters : Outport  Port=2
  Weight Filters : Outport  Port=3
  wires:
  Matrix Concatenation3/1 -> Selector/1
  Data/1 -> Matrix Concatenation3/2, Submatrix1/1
  Selector/1 -> Reshape/1
  Autocorrelation/1 -> Matrix Scaling/1
  LSF Quantization (3.2.4)/2(Quantized LSF Vectors) -> Find Synthesis Filters (3.2.6)/1
  Gain/1 -> Autocorrelation/1
  LSF Quantization (3.2.4)/1(LSF Indices) -> LSF Indices/1
  Reshape/1 -> Gain/1
  Levinson-Durbin/1 -> Matrix Scaling1/1
  Matrix Scaling1/1 -> LPC to LSF/LSP Conversion1/1
  Find Synthesis Filters (3.2.6)/1 -> Synthesis Filters/1
  Find Perceptual Weight Filters (3.2.6)/1 -> Weight Filters/1
  LPC to LSF/LSP Conversion1/1 -> LSF Quantization (3.2.4)/1(LSF Vectors), Find Perceptual Weight Filters (3.2.6)/1
  Matrix Scaling/1 -> Levinson-Durbin/1
  Delay2/1 -> Matrix Concatenation3/1
  Submatrix1/1 -> Delay2/1

== system dspilbclib/iLBC Decoder/Decode Sub-Blocks (4.1 - 4.4)/Decode Remaining Sub-Blocks (4.3 - 4.4) ==
  Initial Codebook : Inport
  Code Indices : Inport  Port=2
  Gain Indices : Inport  Port=3
  Start State Number : Inport  Port=4
  State First : Inport  Port=5
  Compare To Constant2 : simulink/Logic and Bit Operations/Compare To Constant  relop=>  const=0  OutDataTypeStr=uint8  ZeroCross=off
  Decode Remaining Sub-Blocks (4.3 - 4.4) : dspilbclib/Decode Sub-Block  SystemSampleTime=-1  Latency=0  AutoFrameSizeCalculation=off
      settings: SourceProductBaseCode=DS
  For Iterator : ForIterator  ResetStates=reset  IterationLimit=ilbc.NSUB{ilbcMode}-1  IndexMode=Zero-based
  Pad : dspsigops/Pad  padAlong=Columns  dimsToPad=1  valSrc=Specify via dialog  padVal=0  spec=Pad size  padNumOutRowsSpecMethod=User-specified  numOutRows=ilbc.BLOCKL{ilbcMode}-40  padNumOutColsSpecMethod=User-specified  numOutCols=1  isVarDimsMode=off  padBeginning=90  padEnd=0  outSizeMode=User-specified  outSize=1  padSigAt=Beginning  trunc_flag=None  roundingMode=Floor  overflowMode=off  truncOrWrapMode=Truncate  wrap_flag=None
      settings: SourceProductBaseCode=DS
  Selector1 : Selector  NumberOfDimensions=2  IndexMode=Zero-based  InputPortWidth=3  IndexOptions=Select all,Index vector (port)  Indices=-1,0  OutputSizes=1
  Selector3 : Selector  NumberOfDimensions=2  IndexMode=Zero-based  InputPortWidth=3  IndexOptions=Select all,Index vector (port)  Indices=-1,0  OutputSizes=1
  Submatrix : dspmtrx3/Submatrix  RowSpan=Range of rows  RowStartMode=Index  RowStartIndex=41  RowEndMode=Last  RowEndIndex=1  ColSpan=All columns  ColStartMode=First  ColStartIndex=1  ColEndMode=Last  ColEndIndex=1
  Unit Delay External IC : simulink_need_slupdate/Unit Delay External IC  tsamp=-1
      settings: SourceProductBaseCode=SL
  Residual : Outport
  wires:
  For Iterator/1 -> Selector3/2, Compare To Constant2/1, Selector1/2, Decode Remaining Sub-Blocks (4.3 - 4.4)/5
  Decode Remaining Sub-Blocks (4.3 - 4.4)/1 -> Submatrix/1, Residual/1
  Selector3/1 -> Decode Remaining Sub-Blocks (4.3 - 4.4)/3
  Selector1/1 -> Decode Remaining Sub-Blocks (4.3 - 4.4)/4
  Gain Indices/1 -> Selector1/1
  Code Indices/1 -> Selector3/1
  Initial Codebook/1 -> Pad/1
  Submatrix/1 -> Unit Delay External IC/1
  Pad/1 -> Unit Delay External IC/2
  Unit Delay External IC/1 -> Decode Remaining Sub-Blocks (4.3 - 4.4)/1
  Compare To Constant2/1 -> Decode Remaining Sub-Blocks (4.3 - 4.4)/2
  Start State Number/1 -> Decode Remaining Sub-Blocks (4.3 - 4.4)/6
  State First/1 -> Decode Remaining Sub-Blocks (4.3 - 4.4)/7

== system dspilbclib/iLBC Decoder/Decode Sub-Blocks (4.1 - 4.4)/Decoder LPC Analysis (4.1) ==
  LSF Indices : Inport
  Concatenation of Quantized LSFs : Concatenate  NumInputs=3  Mode=Multidimensional array
  Find Synthesis Filters (3.2.6) : dspilbclib/Find LPC Filters  SystemSampleTime=-1  Latency=0  AutoFrameSizeCalculation=off
      settings: SourceProductBaseCode=DS
  Selector3 : Selector  NumberOfDimensions=2  InputPortWidth=3  IndexOptions=Index vector (dialog),Select all  Indices=1,-1  OutputSizes=1
  Selector4 : Selector  NumberOfDimensions=2  InputPortWidth=3  IndexOptions=Index vector (dialog),Select all  Indices=2,-1  OutputSizes=1
  Selector5 : Selector  NumberOfDimensions=2  InputPortWidth=3  IndexOptions=Index vector (dialog),Select all  Indices=3,-1  OutputSizes=1
  Sort : dspstat3/Sort  otype=Value  dir=Ascending  sortAlg=Quick sort  roundingMode=Floor  overflowMode=off
      settings: SourceProductBaseCode=DS
  Vector Quantizer Decoder1 : dspquant2/Vector Quantizer Decoder  invalidin=Clip  CBsource=Specify via dialog  codebook=ilbc.lsfCbTbl1  dataType=Inherit via back propagation  isSigned=on  wordLen=16  udDataType=float('single')  fracBitsMode=Best precision  numFracBits=7  OutDataTypeStr=Inherit: Inherit via back propagation  LastOutDataTypeStr=Inherit: Inherit via back propagation
      settings: SourceProductBaseCode=DS
  Vector Quantizer Decoder2 : dspquant2/Vector Quantizer Decoder  invalidin=Clip  CBsource=Specify via dialog  codebook=ilbc.lsfCbTbl2  dataType=Inherit via back propagation  isSigned=on  wordLen=16  udDataType=float('single')  fracBitsMode=Best precision  numFracBits=7  OutDataTypeStr=Inherit: Inherit via back propagation  LastOutDataTypeStr=Inherit: Inherit via back propagation
      settings: SourceProductBaseCode=DS
  Vector Quantizer Decoder3 : dspquant2/Vector Quantizer Decoder  invalidin=Clip  CBsource=Specify via dialog  codebook=ilbc.lsfCbTbl3  dataType=Inherit via back propagation  isSigned=on  wordLen=16  udDataType=float('single')  fracBitsMode=Best precision  numFracBits=7  OutDataTypeStr=Inherit: Inherit via back propagation  LastOutDataTypeStr=Inherit: Inherit via back propagation
      settings: SourceProductBaseCode=DS
  Synthesis : Outport
  wires:
  LSF Indices/1 -> Selector3/1, Selector4/1, Selector5/1
  Find Synthesis Filters (3.2.6)/1 -> Synthesis/1
  Sort/1 -> Find Synthesis Filters (3.2.6)/1
  Concatenation of Quantized LSFs/1 -> Sort/1
  Vector Quantizer Decoder3/1 -> Concatenation of Quantized LSFs/3
  Vector Quantizer Decoder2/1 -> Concatenation of Quantized LSFs/2
  Vector Quantizer Decoder1/1 -> Concatenation of Quantized LSFs/1
  Selector5/1 -> Vector Quantizer Decoder3/1
  Selector4/1 -> Vector Quantizer Decoder2/1
  Selector3/1 -> Vector Quantizer Decoder1/1

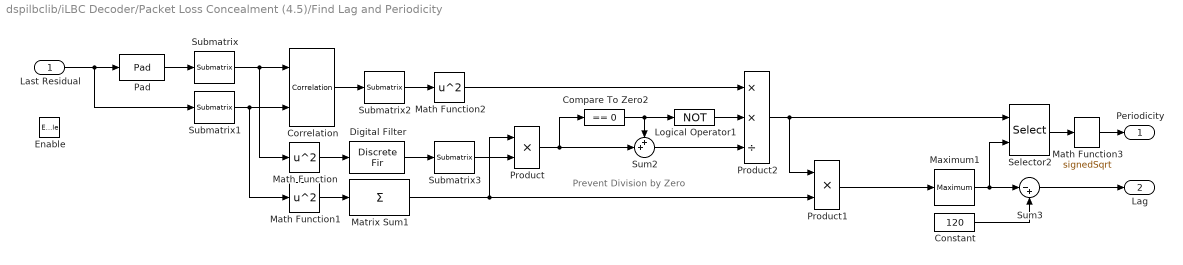
== system dspilbclib/iLBC Decoder/Packet Loss Concealment (4.5)/Find Lag and Periodicity ==
  note: Prevent Division by Zero
  Last Residual : Inport
  Enable : EnablePort
  Compare To Zero2 : simulink/Logic and Bit Operations/Compare To Zero  relop===  OutDataTypeStr=uint8  ZeroCross=off
  Constant : Constant  Value=120  OutDataTypeStr=Inherit: Inherit via back propagation
  Correlation : dspstat3/Correlation  domain=Time  roundingMode=Floor  overflowMode=off  outputDataTypeStr=Inherit: Same as accumulator  outputMin=[]  outputMax=[]  outputLastDataTypeStr=Inherit: Same as accumulator
      settings: SourceProductBaseCode=DS
  Digital Filter : DiscreteFir  Coefficients=(ones(60,1)).'  InputProcessing=Columns as channels (frame based)  AccumDataTypeStr=Inherit: Same as product output
  Logical Operator1 : Logic  Operator=NOT  AllPortsSameDT=off  OutDataTypeStr=boolean
  Math Function : Math  Operator=square  SignedPower=on  SaturateOnIntegerOverflow=on
  Math Function1 : Math  Operator=square  SignedPower=on  SaturateOnIntegerOverflow=on
  Math Function2 : Math  Operator=square  SignedPower=on  SaturateOnIntegerOverflow=on
  Math Function3 : Sqrt  Operator=signedSqrt  AlgorithmType=Newton-Raphson  SaturateOnIntegerOverflow=on
  Matrix Sum1 : Sum  Inputs=+  CollapseMode=Specified dimension  OutDataTypeStr=Inherit: Same as accumulator
  Maximum1 : dspstat3/Maximum  operation=maximum  fcn=Index  indexBase=Zero  operateOver=Each column  Dimension=1  InputProcessing=Columns as channels (frame based)  reset=None  roiEnable=off  roiType=Rectangles  roiPortion=Entire ROI  roiOutput=Individual statistics for each ROI  roiFlag=off  roundingMode=Floor  overflowMode=off  accumDataTypeStr=Inherit: Same as product output  accumLastDataTypeStr=Inherit: Same as product output
  Pad : dspsigops/Pad  padAlong=Columns  dimsToPad=1  valSrc=Specify via dialog  padVal=0  spec=Output size  padNumOutRowsSpecMethod=User-specified  numOutRows=60+120  padNumOutColsSpecMethod=User-specified  numOutCols=1  isVarDimsMode=off  padBeginning=0  padEnd=0  outSizeMode=User-specified  outSize=1  padSigAt=Beginning  trunc_flag=None  roundingMode=Floor  overflowMode=off  truncOrWrapMode=Truncate  wrap_flag=None
      settings: SourceProductBaseCode=DS
  Product : Product  RndMeth=Zero
  Product1 : Product  RndMeth=Zero
  Product2 : Product  Inputs=**/  RndMeth=Zero
  Selector2 : Selector  NumberOfDimensions=2  IndexMode=Zero-based  InputPortWidth=3  IndexOptions=Index vector (port),Index vector (dialog)  Indices=[1 3],0  OutputSizes=7,1
  Submatrix : dspmtrx3/Submatrix  RowSpan=Range of rows  RowStartMode=First  RowStartIndex=120+60-1  RowEndMode=Offset from last  RowEndIndex=20  ColSpan=All columns  ColStartMode=First  ColStartIndex=1  ColEndMode=Last  ColEndIndex=1
  Submatrix1 : dspmtrx3/Submatrix  RowSpan=Range of rows  RowStartMode=Offset from last  RowStartIndex=60-1  RowEndMode=Last  RowEndIndex=60  ColSpan=All columns  ColStartMode=First  ColStartIndex=1  ColEndMode=Last  ColEndIndex=1
  Submatrix2 : dspmtrx3/Submatrix  RowSpan=Range of rows  RowStartMode=Index  RowStartIndex=60  RowEndMode=Offset from last  RowEndIndex=60-1  ColSpan=All columns  ColStartMode=First  ColStartIndex=1  ColEndMode=Last  ColEndIndex=1
  Submatrix3 : dspmtrx3/Submatrix  RowSpan=Range of rows  RowStartMode=Offset from last  RowStartIndex=100  RowEndMode=Last  RowEndIndex=101  ColSpan=All columns  ColStartMode=First  ColStartIndex=1  ColEndMode=Last  ColEndIndex=1
  Sum2 : Sum  Inputs=++|
  Sum3 : Sum  Inputs=|-+
  Periodicity : Outport
  Lag : Outport  Port=2
  wires:
  Compare To Zero2/1 -> Sum2/1, Logical Operator1/1
  Logical Operator1/1 -> Product2/2
  Submatrix3/1 -> Product/2
  Math Function3/1 -> Periodicity/1
  Constant/1 -> Sum3/2
  Product1/1 -> Maximum1/1
  Math Function2/1 -> Product2/1
  Maximum1/1 -> Sum3/1, Selector2/2
  Submatrix/1 -> Correlation/1, Math Function/1
  Submatrix1/1 -> Math Function1/1, Correlation/2
  Sum3/1 -> Lag/1
  Selector2/1 -> Math Function3/1
  Product2/1 -> Selector2/1, Product1/1
  Sum2/1 -> Product2/3
  Product/1 -> Compare To Zero2/1, Sum2/2
  Matrix Sum1/1 -> Product/1, Product1/2
  Digital Filter/1 -> Submatrix3/1
  Math Function/1 -> Digital Filter/1
  Math Function1/1 -> Matrix Sum1/1
  Pad/1 -> Submatrix/1
  Submatrix2/1 -> Math Function2/1
  Correlation/1 -> Submatrix2/1
  Last Residual/1 -> Submatrix1/1, Pad/1
